simulink model "adaptive_dcmotor_2nd_sim"  (R2025b)
settings: Solver=FixedStepDiscrete  StartTime=0.0  StopTime=8  FixedStep=0.002  RelTol=1e-3
model workspace (MAT data in the model file):
  refProfile = [0 0.002 0.004 0.006 0.008 0.01 0.012 0.014 0.016 0.018 0.02 0.022 ... (8002 elements, 4001x2)]
(part 2 of 2)

== matlab function adaptive_dcmotor_2nd_sim/Adaptive RST controller/Pole placement ==
  data: a1 input; c0 output; a0 input; b1 input; b0 input; q0 input; q1 input; q2 input; q3 input; kFreeze input; d2 output; d1 output; d0 output
function [c0,d2,d1,d0] = pole_placement(a1,a0,b1,b0,q0,q1,q2,q3,kFreeze)
                                                                       %#codegen                                                               
                                                                       % From (z^2+a1*z+a0)(z-1)(z+c0) +                                       
                                                                       % (b1*z+b0)(d2*z^2+d1*z+d0) = z^4+q3*z^3+q2*z^2+q1*z+q0.                
                                                                       % Matching z^3..z^0 coefficients gives M*[c0; d2; d1; d0] = rhs.        
                                                                       persistent c0Hold d2Hold d1Hold d0Hold k                                
                                                                       if isempty(k)                                                           
                                                                           c0Hold = 0.0;                                                       
                                                                           d2Hold = 0.2;                                                       
                                                                           d1Hold = 0.0;                                                       
                                                                           d0Hold = 0.0;                                                       
                                                                           k = 0.0;                                                            
                                                                       end                                                                     
                                                                       if k >= kFreeze                                                         
                                                                           M = [1.0,     b1, 0.0, 0.0;                                         
                                                                                a1-1.0,  b0, b1,  0.0;                                         
                                                                                a0-a1,  0.0, b0,  b1;                                          
                                                                               -a0,     0.0, 0.0, b0];                                         
                                                                           rhs = [q3 - a1 + 1.0; q2 - a0 + a1; q1 + a0; q0];                   
                                                                           if rcond(M) >= 1e-8                                                 
                                                                               sol = M \ rhs;                                                  
                                                                               if all(isfinite(sol))                                           
                                                                                   c0Hold = sol(1);                                            
                                                                                   d2Hold = sol(2);                                            
                                                                                   d1Hold = sol(3);                                            
                                                                                   d0Hold = sol(4);                                            
                                                                               end                                                             
                                                                           end                                                                 
                                                                       end                                                                     
                                                                       k = k + 1.0;                                                            
                                                                       c0 = c0Hold;                                                            
                                                                       d2 = d2Hold;                                                            
                                                                       d1 = d1Hold;                                                            
                                                                       d0 = d0Hold;                                                            
                                                                       end

== matlab function adaptive_dcmotor_2nd_sim/Adaptive RST controller/RLS Estimator ==
  data: y input; a1_est output; y1 input; y2 input; u1 input; u2 input; alpha input; a0_est output; b1_est output; b0_est output; traceP output
function [a1_est,a0_est,b1_est,b0_est,traceP] = rls_estimator(y,y1,y2,u1,u2,alpha)                  
                                                                                                   %#codegen                                                                                           
                                                                                                   % RLS for y(k) = [-y(k-1), -y(k-2), u(k-1), u(k-2)] * theta.                                        
                                                                                                   % Use alpha = 1 here; alpha < 1 without persistent excitation causes covariance windup and bursting.
                                                                                                   % The excitation gate skips idle updates, and the trace limit is a final guard.                     
                                                                                                   persistent P theta                                                                                  
                                                                                                   if isempty(P)                                                                                       
                                                                                                       P =                                                                                             100                                                                                                  * eye(4);                                                                                          
                                                                                                       theta = [-1.0; 0.2; 0.05; 0.02];                                                                
                                                                                                   end                                                                                                 
                                                                                                   phi = [-y1; -y2; u1; u2];                                                                           
                                                                                                   if (phi' * phi) > 1e-8                                                                              
                                                                                                       den = phi' * P * phi + alpha;                                                                   
                                                                                                       L = (P * phi) / den;                                                                            
                                                                                                       thetaNew = theta + L * (y - phi' * theta);                                                      
                                                                                                       PNew = (eye(4) - L * phi') * P / alpha;                                                         
                                                                                                       PNew = 0.5 * (PNew + PNew');                                                                    
                                                                                                       trNew = trace(PNew);                                                                            
                                                                                                       if isfinite(trNew) && all(isfinite(thetaNew))                                                   
                                                                                                           theta = thetaNew;                                                                           
                                                                                                           P = PNew;                                                                                   
                                                                                                       end                                                                                             
                                                                                                   end                                                                                                 
                                                                                                   tr = trace(P);                                                                                      
                                                                                                   if tr >                                                                                             9000                                                                                                
                                                                                                       P = P * (                                                                                       9000                                                                                                 / tr);                                                                                             
                                                                                                       tr = trace(P);                                                                                  
                                                                                                   end                                                                                                 
                                                                                                   a1_est = theta(1);                                                                                  
                                                                                                   a0_est = theta(2);                                                                                  
                                                                                                   b1_est = theta(3);                                                                                  
                                                                                                   b0_est = theta(4);                                                                                  
                                                                                                   traceP = tr;                                                                                        
                                                                                                   end

== matlab function adaptive_dcmotor_2nd_sim/Adaptive RST controller/RST law ==
  data: c0 input; u output; d2 input; d1 input; d0 input; e input; e1 input; e2 input; u1 input; u2 input
function u = rst_law(c0,d2,d1,d0,e,e1,e2,u1,u2)                    
                                                                  %#codegen                                                          
                                                                  % Gc(z)=D(z)/((z-1)(z+c0)); divide by z^2 to obtain this recursion.
                                                                  u = u1 - c0 * (u1 - u2) + d2 * e + d1 * e1 + d0 * e2;              
                                                                  end
